simulink model "refModel"  (R2014a)
settings: Solver=ode1  StartTime=0.0  StopTime=10.0  FixedStep=0.1  RelTol=1e-3
settings Model: Creator=mbrauer  LastModifiedBy=mbrauer

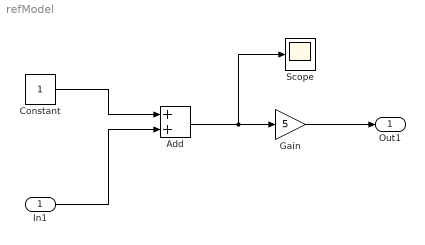
== system refModel ==
  In1 : Inport
  Add : Sum
  Constant : Constant
  Gain : Gain  Gain=5
  Scope : Scope
  Out1 : Outport
  wires:
  Constant/1 -> Add/1
  In1/1 -> Add/2
  Add/1 -> Scope/1, Gain/1
  Gain/1 -> Out1/1
